simulink model "item4ModeloNLinPS"  (R2018a)
settings: Solver=VariableStepAuto  StartTime=0.0  StopTime=100  RelTol=1e-3
values from neighbouring files (symbols this model uses):
  C_d = minreal(c2d(C, Ts, 'matched'))    [psfRapido.m]    (also in psfRapido_IMC.m)
  F_d = minreal(c2d(F, Ts, 'matched'))    [psfRapido.m]    (also in psfRapido_IMC.m)
  Fr = minreal(NumFr/DenFr)    [psfRapido.m]    (also in psfRapido_IMC.m)
  Gu_d = minreal(c2d(Gu, Ts, 'zoh'))    [psfRapido.m]    (also in psfRapido_IMC.m)
  Kc = (1/(2*L))*(1/(Ke/Ti))    (= 0.102221616464)    [Analise_robustez_q4.m]    (also in psfRapido.m; psfRapido_IMC.m; scriptAux.m)
  Td = t2    (= 0.2)    [Analise_robustez_q4.m]    (also in psfRapido.m; psfRapido_IMC.m; scriptAux.m)
  Ti = t1    (= 0.45)    [Analise_robustez_q4.m]    (also in psfRapido.m; psfRapido_IMC.m; scriptAux.m)
  Ts = t_5/20    (= 0.075)    [psfRapido.m]    (also in psfRapido_IMC.m)
libraries: simulink x4
settings Model: Creator=julia  LastModifiedBy=crist
settings CodeAppCC: StateflowObjectComments=on

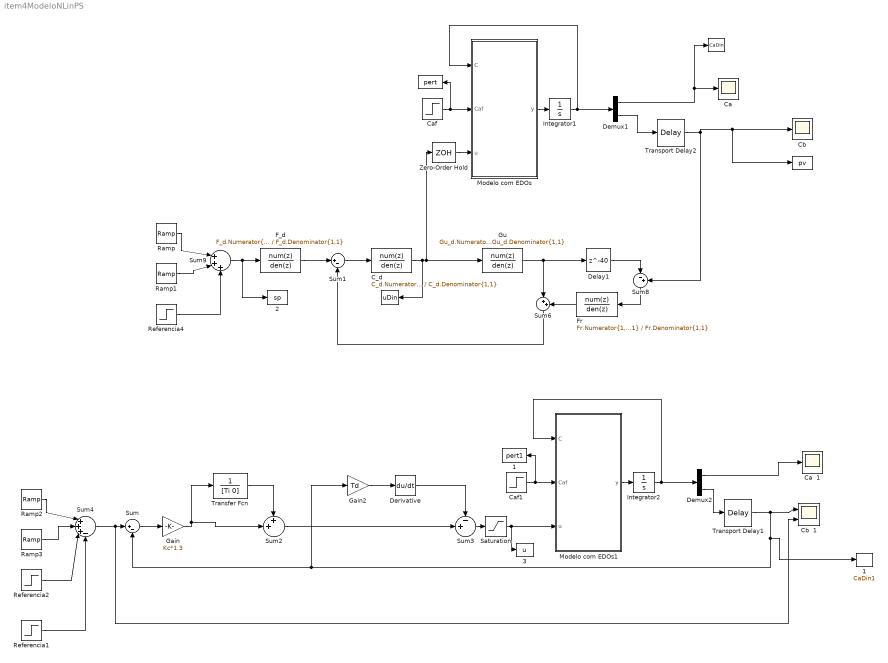
== system item4ModeloNLinPS ==
  "   " : ToWorkspace  VariableName=pv  SaveFormat=Timeseries  SampleTime=-1
  "          " : ToWorkspace  VariableName=pert  SaveFormat=Timeseries  SampleTime=-1
  "                 " : ToWorkspace  VariableName=uDin  SaveFormat=Timeseries  SampleTime=-1
  "                   " : ToWorkspace  VariableName=CaDin  SaveFormat=Timeseries  SampleTime=-1
  "                   1" : ToWorkspace  VariableName=CaDin1  SaveFormat=Timeseries  SampleTime=-1
  "                   3" : ToWorkspace  VariableName=u  SaveFormat=Timeseries  SampleTime=-1
  "          1" : ToWorkspace  VariableName=pert1  SaveFormat=Timeseries  SampleTime=-1
  "   2" : ToWorkspace  VariableName=sp  SaveFormat=Timeseries  SampleTime=-1
  C_d : DiscreteTransferFcn  Numerator=C_d.Numerator{1,1}  Denominator=C_d.Denominator{1,1}  SampleTime=Ts
  "Ca  " : Scope
  Ca  1 : Scope
  Caf : Step  Time=60  Before=5.1  After=5.15  SampleTime=0
  Caf1 : Step  Time=180  Before=5.1  After=5.2  SampleTime=0
  "Cb  " : Scope
  Cb  1 : Scope  NumInputPorts=2
  Delay1 : Delay  DelayLength=40  InitialCondition=0
  Demux1 : Demux  Outputs=2
  Demux2 : Demux  Outputs=2
  Derivative : Derivative
  F_d : DiscreteTransferFcn  Numerator=F_d.Numerator{1,1}  Denominator=F_d.Denominator{1,1}  SampleTime=Ts
  Fr : DiscreteTransferFcn  Numerator=Fr.Numerator{1,1}  Denominator=Fr.Denominator{1,1}  SampleTime=Ts
  Gain : Gain  Gain=Kc*1.3
  Gain2 : Gain  Gain=Td
  "Gu " : DiscreteTransferFcn  Numerator=Gu_d.Numerator{1,1}  Denominator=Gu_d.Denominator{1,1}  SampleTime=Ts
  Integrator1 : Integrator  InitialCondition=[0;0]
  Integrator2 : Integrator  InitialCondition=[0;0]
  Modelo com EDOs : MATLAB Function  TreatAsAtomicUnit=on
  Modelo com EDOs1 : MATLAB Function  TreatAsAtomicUnit=on
  Ramp : simulink/Sources/Ramp  slope=2.345/10  start=0  InitialOutput=0
  Ramp1 : simulink/Sources/Ramp  slope=-2.345/10  start=10  InitialOutput=0
  Ramp2 : simulink/Sources/Ramp  slope=2.345/50  start=0  InitialOutput=0
  Ramp3 : simulink/Sources/Ramp  slope=-2.345/50  start=50  InitialOutput=0
  Referencia1 : Step  Time=140  After=0  SampleTime=0
  Referencia2 : Step  Time=130  After=0.25  SampleTime=0
  Referencia4 : Step  Time=30  After=0.1  SampleTime=0
  Saturation : Saturate  UpperLimit=5  LowerLimit=0
  Sum : Sum  Inputs=|+-
  Sum1 : Sum  Inputs=|+-
  Sum2 : Sum  Inputs=++|
  Sum3 : Sum  Inputs=-+|
  Sum4 : Sum  Inputs=|+++-
  Sum6 : Sum  Inputs=|++
  Sum8 : Sum  Inputs=|-+
  Sum9 : Sum  Inputs=|+++
  Transfer Fcn : TransferFcn  Denominator=[Ti 0]
  Transport Delay1 : TransportDelay  DelayTime=3
  Transport Delay2 : TransportDelay  DelayTime=3
  Zero-Order Hold : ZeroOrderHold  SampleTime=-1
  wires:
  Modelo com EDOs/1(y) -> Integrator1/1
  Integrator1/1 -> Modelo com EDOs/1(C), Demux1/1
  Demux1/1 -> "                   "/1, "Ca  "/1
  Caf/1 -> "          "/1, Modelo com EDOs/2(Caf)
  Referencia4/1 -> Sum9/3
  Ramp1/1 -> Sum9/2
  Ramp/1 -> Sum9/1
  Demux1/2 -> Transport Delay2/1
  F_d/1 -> Sum1/1
  Sum8/1 -> Fr/1
  Sum6/1 -> Sum1/2
  C_d/1 -> "                 "/1, Zero-Order Hold/1, "Gu "/1
  Sum9/1 -> "   2"/1, F_d/1
  Fr/1 -> Sum6/2
  "Gu "/1 -> Sum6/1, Delay1/1
  Delay1/1 -> Sum8/1
  Sum1/1 -> C_d/1
  Transport Delay2/1 -> "   "/1, "Cb  "/1, Sum8/2
  Saturation/1 -> Modelo com EDOs1/3(u), "                   3"/1
  Derivative/1 -> Sum3/1
  Ramp2/1 -> Sum4/1
  Referencia1/1 -> Sum4/4
  Demux2/1 -> Ca  1/1
  Sum/1 -> Gain/1
  Integrator2/1 -> Modelo com EDOs1/1(C), Demux2/1
  Gain2/1 -> Derivative/1
  Referencia2/1 -> Sum4/3
  Sum3/1 -> Saturation/1
  Demux2/2 -> Transport Delay1/1
  Modelo com EDOs1/1(y) -> Integrator2/1
  Gain/1 -> Sum2/2, Transfer Fcn/1
  Sum2/1 -> Sum3/2
  Caf1/1 -> "          1"/1, Modelo com EDOs1/2(Caf)
  Transport Delay1/1 -> "                   1"/1, Sum/2, Gain2/1, Cb  1/1
  Sum4/1 -> Sum/1, Cb  1/2
  Ramp3/1 -> Sum4/2
  Transfer Fcn/1 -> Sum2/1
  Zero-Order Hold/1 -> Modelo com EDOs/3(u)

== matlab function item4ModeloNLinPS/Modelo com EDOs ==
  data: y output; C input; Caf input; u input
%EDOs das concentracoes dos produtos A e B
function y = fcn(C, Caf, u)

%constantes
k1 = 6.01; %L/min
k2 = 0.8433; %L/min
k3 = 0.1123; %mol/Lmin

%variaveis das concentracoes dos produtos A e B
Ca = C(1);
Cb = C(2);

%EDOs
Ca_d = -k1*Ca - k3*(Ca^2) + (Caf - Ca)*u;
Cb_d =  k1*Ca - k2*Cb - Cb*u;
 
%conjunto das EDOs
y = [Ca_d;Cb_d];

== matlab function item4ModeloNLinPS/Modelo com EDOs1 ==
  data: y output; C input; Caf input; u input
%EDOs das concentracoes dos produtos A e B
function y = fcn(C, Caf, u)

%constantes
k1 = 6.01; %L/min
k2 = 0.8433; %L/min
k3 = 0.1123; %mol/Lmin

%variaveis das concentracoes dos produtos A e B
Ca = C(1);
Cb = C(2);

%EDOs
Ca_d = -k1*Ca - k3*(Ca^2) + (Caf - Ca)*u;
Cb_d =  k1*Ca - k2*Cb - Cb*u;
 
%conjunto das EDOs
y = [Ca_d;Cb_d];
